simulink library "lib_cosimulation"  (Simulink 4.1.1)
undefined symbols (not defined in the file or in its folder): acc_elec_eff, acc_elec_pwr, ess2_ah_nom_fun, ess2_cap_scale, ess2_dcdc_curroutmax, ess2_dcdc_eff, ess2_dcdc_vmaxout_fun, ess2_dcdc_vminin_fun, ess2_dcdc_vminout_fun, ess2_fah_max, ess2_fah_thi, ess2_fc, ess2_init_soc, ess2_max_volts, ess2_min_volts, ess2_module_num, ess2_rnom, ess2_self_disc, ess2_sg_disc, ess2_sg_full, ess2_SOC2sg, ess2_voc, ess_ah_nom_fun, ess_cap_scale, ess_fah_max, ess_fah_thi, ess_fc, ess_init_soc, ess_max_volts, ess_min_volts, ess_module_num, ess_rnom, ess_self_disc, ess_sg_disc, ess_sg_full, ess_SOC2sg, ess_voc, fc_on, gc_cutin12, gc_cutin93, gc_eff, gc_inertia, gc_map_spd, gc_max_crrnt, gc_min_volts, gc_spd_scale, gc_t12, gc_t93, gc_tempalt, gc_user_imax12, gc_user_imax93, gc_vehicletype, mc_inertia, mc_map_spd, mc_max_crrnt, mc_min_volts, mc_spd_scale, reg_temp1, reg_temp2, reg_tempreg ... (+7)
libraries: lib_cosimulation x20
(part 1 of 2)
settings Model: LastModifiedBy=abrooker
settings Model: ModifiedHistory=|
  | [mokeefe] 22-April-2002
  | In 14V Load Control/Starter, added a memory block after the eng_on FROM tag with initial condition equal to fc_on

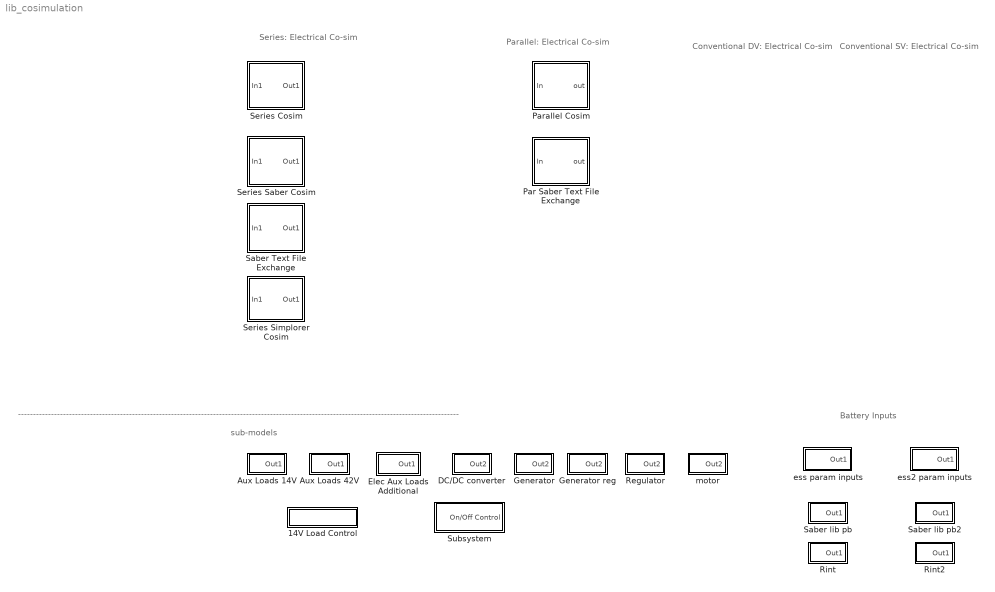
== system lib_cosimulation ==
  note: Series: Electrical Co-sim
  note: Conventional DV:
      | Electrical Co-sim
  note: ---------------------------------------------------------------------------------------------------------------------------------------------------
  note: sub-models
  note: Conventional SV:
      | Electrical Co-sim
  note: Parallel: Electrical Co-sim
  note: Battery Inputs
  14V Load Control : Subsystem
      settings: RTWFcnNameOpts=Auto  RTWFileNameOpts=Auto
  Aux Loads 14V : Subsystem
      settings: RTWFcnNameOpts=Auto  RTWFileNameOpts=Auto
  Aux Loads 42V : Subsystem
      settings: RTWFcnNameOpts=Auto  RTWFileNameOpts=Auto
  DC/DC converter : Subsystem
      settings: RTWFcnNameOpts=Auto  RTWFileNameOpts=Auto
  Elec Aux Loads Additional : Subsystem
      settings: RTWFcnNameOpts=Auto  RTWFileNameOpts=Auto
  Generator : Subsystem
      settings: RTWFcnNameOpts=Auto  RTWFileNameOpts=Auto
  Generator reg : Subsystem
      settings: RTWFcnNameOpts=Auto  RTWFileNameOpts=Auto
  Par Saber Text File Exchange : Subsystem
      settings: RTWFcnNameOpts=Auto  RTWFileNameOpts=Auto
      mask Display: image(imread('saber.bmp'))
  Parallel Cosim : Subsystem  BlockChoice=Par Saber Text File Exchange
      settings: TemplateBlock=self  MemberBlocks=Par Saber Text File Exchange  RTWFcnNameOpts=Auto  RTWFileNameOpts=Auto
  Regulator : Subsystem
      settings: RTWFcnNameOpts=Auto  RTWFileNameOpts=Auto
  Rint : Subsystem
      settings: RTWFcnNameOpts=Auto  RTWFileNameOpts=Auto
  Rint2 : Subsystem
      settings: RTWFcnNameOpts=Auto  RTWFileNameOpts=Auto
  Saber Text File Exchange : Subsystem  AncestorBlock=lib_cosimulation/SaberCosim
      settings: RTWFcnNameOpts=Auto  RTWFileNameOpts=Auto
      mask Display: image(imread('saber.bmp'))
  Saber lib pb : Subsystem
      settings: RTWFcnNameOpts=Auto  RTWFileNameOpts=Auto
  Saber lib pb2 : Subsystem
      settings: RTWFcnNameOpts=Auto  RTWFileNameOpts=Auto
  Series Cosim : Subsystem  BlockChoice=Series Saber Cosim
      settings: TemplateBlock=self  MemberBlocks=Saber Text File Exchange,Series Saber Cosim,Series Simplorer Cosim  RTWFcnNameOpts=Auto  RTWFileNameOpts=Auto
  Series Saber Cosim : Subsystem
      settings: RTWFcnNameOpts=Auto  RTWFileNameOpts=Auto
      mask Display: image(imread('saber.bmp'))
  Series Simplorer Cosim : Subsystem  AncestorBlock=lib_cosimulation/SaberCosim
      settings: RTWFcnNameOpts=Auto  RTWFileNameOpts=Auto
      mask Display: image(imread('simplorer.bmp'))
  Subsystem : Subsystem  mask{ModelName='Radio'}
      mask prompts: ModelName "Load Name (example: 'Radio')"
      settings: RTWFcnNameOpts=Auto  RTWFileNameOpts=Auto
  ess param inputs : Subsystem  BlockChoice=Rint
      settings: TemplateBlock=self  MemberBlocks=Rint,Saber lib pb  RTWFcnNameOpts=Auto  RTWFileNameOpts=Auto
  ess2 param inputs : Subsystem  BlockChoice=Rint2
      settings: TemplateBlock=self  MemberBlocks=Rint2,Saber lib pb2  RTWFcnNameOpts=Auto  RTWFileNameOpts=Auto
  motor : Subsystem
      settings: RTWFcnNameOpts=Auto  RTWFileNameOpts=Auto

== system lib_cosimulation/14V Load Control ==
  Starter : Subsystem
      settings: RTWFcnNameOpts=Auto  RTWFileNameOpts=Auto

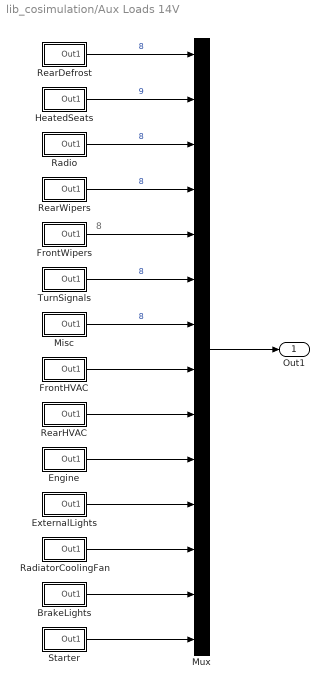
== system lib_cosimulation/Aux Loads 14V ==
  note: 8
  BrakeLights : Subsystem
      settings: RTWFcnNameOpts=Auto  RTWFileNameOpts=Auto
  Engine : Subsystem
      settings: RTWFcnNameOpts=Auto  RTWFileNameOpts=Auto
  ExternalLights : Subsystem
      settings: RTWFcnNameOpts=Auto  RTWFileNameOpts=Auto
  FrontHVAC : Subsystem
      settings: RTWFcnNameOpts=Auto  RTWFileNameOpts=Auto
  FrontWipers : Subsystem
      settings: RTWFcnNameOpts=Auto  RTWFileNameOpts=Auto
  HeatedSeats : Subsystem
      settings: RTWFcnNameOpts=Auto  RTWFileNameOpts=Auto
  Misc : Subsystem
      settings: RTWFcnNameOpts=Auto  RTWFileNameOpts=Auto
  Mux : Mux  Inputs=14
  RadiatorCoolingFan : Subsystem
      settings: RTWFcnNameOpts=Auto  RTWFileNameOpts=Auto
  Radio : Subsystem
      settings: RTWFcnNameOpts=Auto  RTWFileNameOpts=Auto
  RearDefrost : Subsystem
      settings: RTWFcnNameOpts=Auto  RTWFileNameOpts=Auto
  RearHVAC : Subsystem
      settings: RTWFcnNameOpts=Auto  RTWFileNameOpts=Auto
  RearWipers : Subsystem
      settings: RTWFcnNameOpts=Auto  RTWFileNameOpts=Auto
  Starter : Subsystem
      settings: RTWFcnNameOpts=Auto  RTWFileNameOpts=Auto
  TurnSignals : Subsystem
      settings: RTWFcnNameOpts=Auto  RTWFileNameOpts=Auto
  Out1 : Outport  Port=1
  wires:
  BrakeLights/1(Out1) -> Mux/13
  RadiatorCoolingFan/1(Out1) -> Mux/12
  ExternalLights/1(Out1) -> Mux/11
  Engine/1(Out1) -> Mux/10
  RearHVAC/1(Out1) -> Mux/9
  FrontHVAC/1(Out1) -> Mux/8
  Misc/1(Out1) -> Mux/7  "8"
  TurnSignals/1(Out1) -> Mux/6  "8"
  FrontWipers/1(Out1) -> Mux/5
  RearWipers/1(Out1) -> Mux/4  "8"
  Radio/1(Out1) -> Mux/3  "8"
  HeatedSeats/1(Out1) -> Mux/2  "9"
  RearDefrost/1(Out1) -> Mux/1  "8"
  Mux/1 -> Out1/1
  Starter/1(Out1) -> Mux/14

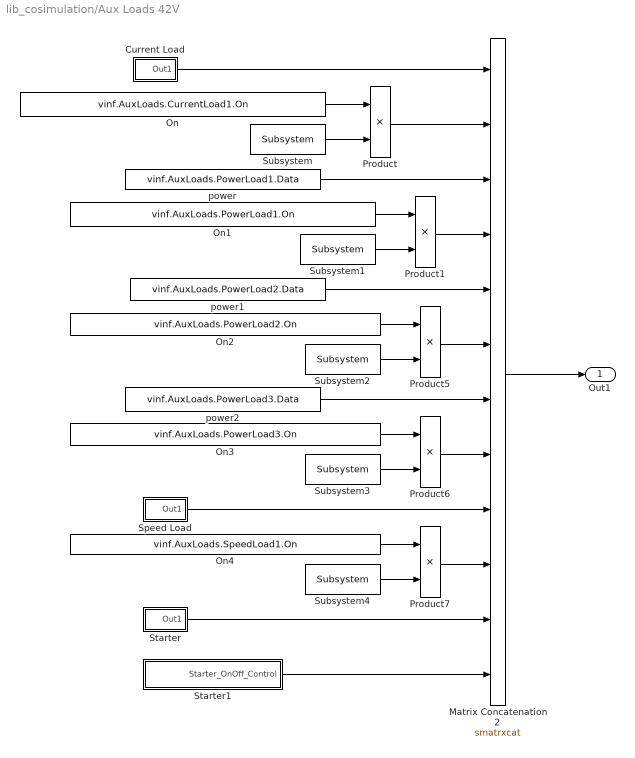
== system lib_cosimulation/Aux Loads 42V ==
  Current Load : Subsystem
      settings: RTWFcnNameOpts=Auto  RTWFileNameOpts=Auto
  Matrix Concatenation2 : S-Function  FunctionName=smatrxcat  Parameters=numInports,catMethod  PortCounts=[]  SFunctionModules=''  mask(Matrix Concatenation){numInports=12, catMethod=Horizontal}
      mask prompts: numInports "Number of inputs:"; catMethod "Concatenation method:"
      mask help: Perform horizontal or vertical concatenation. 1-D vector input signals are treated as column vectors, i.e., [Mx1] matrices. The output is always a matrix.
      mask init:
      | xy = matrxcatmask('icon');
      mask StyleString: edit,popup(Horizontal|Vertical)
      mask Display:
      | plot(xy.x,xy.y);
      | text(0.15,0.86,xy.label);
  On : Constant  Value=vinf.AuxLoads.CurrentLoad1.On
  On1 : Constant  Value=vinf.AuxLoads.PowerLoad1.On
  On2 : Constant  Value=vinf.AuxLoads.PowerLoad2.On
  On3 : Constant  Value=vinf.AuxLoads.PowerLoad3.On
  On4 : Constant  Value=vinf.AuxLoads.SpeedLoad1.On
  Product{,1,5..7} (5 alike) : Product  Inputs=2  Multiplication=Element-wise(.*)  SaturateOnIntegerOverflow=on
  Speed Load : Subsystem
      settings: RTWFcnNameOpts=Auto  RTWFileNameOpts=Auto
  Starter : Subsystem
      settings: RTWFcnNameOpts=Auto  RTWFileNameOpts=Auto
  Starter1 : Subsystem
      settings: RTWFcnNameOpts=Auto  RTWFileNameOpts=Auto
  Subsystem : lib_cosimulation/Subsystem  ModelName='CurrentLoad1'
  Subsystem1 : lib_cosimulation/Subsystem  ModelName='PowerLoad1'
  Subsystem2 : lib_cosimulation/Subsystem  ModelName='PowerLoad2'
  Subsystem3 : lib_cosimulation/Subsystem  ModelName='PowerLoad3'
  Subsystem4 : lib_cosimulation/Subsystem  ModelName='SpeedLoad1'
  power : Constant  Value=vinf.AuxLoads.PowerLoad1.Data
  power1 : Constant  Value=vinf.AuxLoads.PowerLoad2.Data
  power2 : Constant  Value=vinf.AuxLoads.PowerLoad3.Data
  Out1 : Outport  Port=1
  wires:
  power1/1 -> Matrix Concatenation2/5
  power/1 -> Matrix Concatenation2/3
  Matrix Concatenation2/1 -> Out1/1
  Speed Load/1(Out1) -> Matrix Concatenation2/9
  Current Load/1(Out1) -> Matrix Concatenation2/1
  Starter/1(Out1) -> Matrix Concatenation2/11
  power2/1 -> Matrix Concatenation2/7
  Product/1 -> Matrix Concatenation2/2
  On/1 -> Product/1
  Subsystem/1 -> Product/2
  On1/1 -> Product1/1
  Subsystem1/1 -> Product1/2
  Product1/1 -> Matrix Concatenation2/4
  Product5/1 -> Matrix Concatenation2/6
  On2/1 -> Product5/1
  Subsystem2/1 -> Product5/2
  Product6/1 -> Matrix Concatenation2/8
  On3/1 -> Product6/1
  Subsystem3/1 -> Product6/2
  Product7/1 -> Matrix Concatenation2/10
  Subsystem4/1 -> Product7/2
  On4/1 -> Product7/1
  Starter1/1(Starter_OnOff_Control) -> Matrix Concatenation2/12

== system lib_cosimulation/DC/DC converter ==
  Constant1 : Constant  Value=ess2_dcdc_eff
  Constant4 : Constant  Value=ess2_dcdc_curroutmax
  Matrix Concatenation1 : S-Function  FunctionName=smatrxcat  Parameters=numInports,catMethod  PortCounts=[]  SFunctionModules=''  mask(Matrix Concatenation){numInports=6, catMethod=Horizontal}
      mask prompts: numInports "Number of inputs:"; catMethod "Concatenation method:"
      mask help: Perform horizontal or vertical concatenation. 1-D vector input signals are treated as column vectors, i.e., [Mx1] matrices. The output is always a matrix.
      mask init:
      | xy = matrxcatmask('icon');
      mask StyleString: edit,popup(Horizontal|Vertical)
      mask Display:
      | plot(xy.x,xy.y);
      | text(0.15,0.86,xy.label);
  ess2_dcdc_vmaxout : Constant  Value=ess2_dcdc_vmaxout_fun(0)
  ess2_dcdc_vminin : Constant  Value=ess2_dcdc_vminin_fun(0)
  ess2_dcdc_vminout : Constant  Value=ess2_dcdc_vminout_fun(0)
  Out2 : Outport  Port=1
  wires:
  Matrix Concatenation1/1 -> Out2/1
  [key_on] -> Matrix Concatenation1/1
  Constant1/1 -> Matrix Concatenation1/2
  ess2_dcdc_vminout/1 -> Matrix Concatenation1/3
  ess2_dcdc_vmaxout/1 -> Matrix Concatenation1/4
  Constant4/1 -> Matrix Concatenation1/5
  ess2_dcdc_vminin/1 -> Matrix Concatenation1/6

== system lib_cosimulation/Elec Aux Loads Additional ==
  Constant : Constant  Value=acc_elec_pwr
  Product : Product  Inputs=2  Multiplication=Element-wise(.*)  SaturateOnIntegerOverflow=on
  eff : Gain  Gain=1/acc_elec_eff  Multiplication=Element-wise(K.*u)  SaturateOnIntegerOverflow=on
  Out1 : Outport  Port=1
  wires:
  Product/1 -> Out1/1
  [key_on] -> Product/1
  eff/1 -> Product/2
  Constant/1 -> eff/1

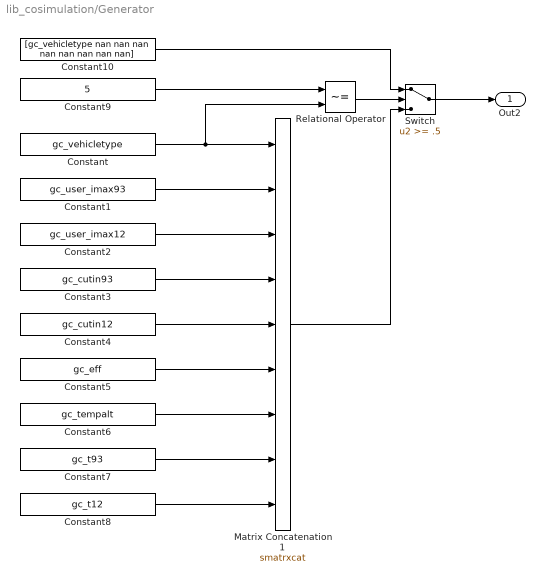
== system lib_cosimulation/Generator ==
  Constant : Constant  Value=gc_vehicletype
  Constant1 : Constant  Value=gc_user_imax93
  Constant10 : Constant  Value=[gc_vehicletype nan nan nan nan nan nan nan nan]
  Constant2 : Constant  Value=gc_user_imax12
  Constant3 : Constant  Value=gc_cutin93
  Constant4 : Constant  Value=gc_cutin12
  Constant5 : Constant  Value=gc_eff
  Constant6 : Constant  Value=gc_tempalt
  Constant7 : Constant  Value=gc_t93
  Constant8 : Constant  Value=gc_t12
  Constant9 : Constant  Value=5
  Matrix Concatenation1 : S-Function  FunctionName=smatrxcat  Parameters=numInports,catMethod  PortCounts=[]  SFunctionModules=''  mask(Matrix Concatenation){numInports=9, catMethod=Horizontal}
      mask prompts: numInports "Number of inputs:"; catMethod "Concatenation method:"
      mask help: Perform horizontal or vertical concatenation. 1-D vector input signals are treated as column vectors, i.e., [Mx1] matrices. The output is always a matrix.
      mask init:
      | xy = matrxcatmask('icon');
      mask StyleString: edit,popup(Horizontal|Vertical)
      mask Display:
      | plot(xy.x,xy.y);
      | text(0.15,0.86,xy.label);
  Relational Operator : RelationalOperator  Operator=~=
  Switch : Switch  Threshold=.5
  Out2 : Outport  Port=1
  wires:
  Constant8/1 -> Matrix Concatenation1/9
  Switch/1 -> Out2/1
  Constant1/1 -> Matrix Concatenation1/2
  Constant2/1 -> Matrix Concatenation1/3
  Constant3/1 -> Matrix Concatenation1/4
  Constant4/1 -> Matrix Concatenation1/5
  Constant5/1 -> Matrix Concatenation1/6
  Constant6/1 -> Matrix Concatenation1/7
  Constant7/1 -> Matrix Concatenation1/8
  Relational Operator/1 -> Switch/2
  Matrix Concatenation1/1 -> Switch/3
  Constant9/1 -> Relational Operator/1
  Constant/1 -> Matrix Concatenation1/1, Relational Operator/2
  Constant10/1 -> Switch/1

== system lib_cosimulation/Generator reg ==
  Constant5 : Constant  Value=gc_inertia
  Constant7 : Constant  Value=gc_max_crrnt
  Constant8 : Constant  Value=gc_min_volts
  Matrix Concatenation1 : S-Function  FunctionName=smatrxcat  Parameters=numInports,catMethod  PortCounts=[]  SFunctionModules=''  mask(Matrix Concatenation){numInports=4, catMethod=Horizontal}
      mask prompts: numInports "Number of inputs:"; catMethod "Concatenation method:"
      mask help: Perform horizontal or vertical concatenation. 1-D vector input signals are treated as column vectors, i.e., [Mx1] matrices. The output is always a matrix.
      mask init:
      | xy = matrxcatmask('icon');
      mask StyleString: edit,popup(Horizontal|Vertical)
      mask Display:
      | plot(xy.x,xy.y);
      | text(0.15,0.86,xy.label);
  max gc spd : Constant  Value=max(gc_map_spd)*gc_spd_scale
  Out2 : Outport  Port=1
  wires:
  Constant7/1 -> Matrix Concatenation1/3
  max gc spd/1 -> Matrix Concatenation1/2
  Constant5/1 -> Matrix Concatenation1/1
  Constant8/1 -> Matrix Concatenation1/4
  Matrix Concatenation1/1 -> Out2/1

== system lib_cosimulation/Par Saber Text File Exchange ==
  In : Inport  Port=1  LatchInput=off
  S-Function that calls  Saber co-simulation1 : S-Function  FunctionName=SaberCosimSfun  Parameters=vinf.tmppath,time_step,['SaberCosimIO_PAR']  PortCounts=[]  SFunctionModules=''
  out : Outport  Port=1
  wires:
  In/1 -> S-Function that calls  Saber co-simulation1/1
  S-Function that calls  Saber co-simulation1/1 -> out/1

== system lib_cosimulation/Parallel Cosim ==
  In : Inport  Port=1  LatchInput=off
  Par Saber Text File Exchange : lib_cosimulation/Par Saber Text File Exchange
  out : Outport  Port=1
  wires:
  In/1 -> Par Saber Text File Exchange/1
  Par Saber Text File Exchange/1 -> out/1

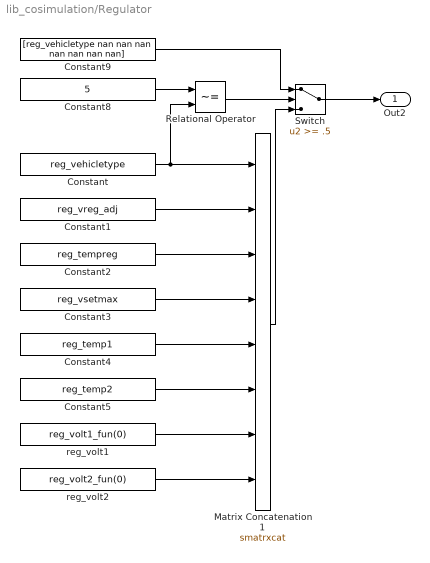
== system lib_cosimulation/Regulator ==
  Constant : Constant  Value=reg_vehicletype
  Constant1 : Constant  Value=reg_vreg_adj
  Constant2 : Constant  Value=reg_tempreg
  Constant3 : Constant  Value=reg_vsetmax
  Constant4 : Constant  Value=reg_temp1
  Constant5 : Constant  Value=reg_temp2
  Constant8 : Constant  Value=5
  Constant9 : Constant  Value=[reg_vehicletype nan nan nan nan nan nan nan]
  Matrix Concatenation1 : S-Function  FunctionName=smatrxcat  Parameters=numInports,catMethod  PortCounts=[]  SFunctionModules=''  mask(Matrix Concatenation){numInports=8, catMethod=Horizontal}
      mask prompts: numInports "Number of inputs:"; catMethod "Concatenation method:"
      mask help: Perform horizontal or vertical concatenation. 1-D vector input signals are treated as column vectors, i.e., [Mx1] matrices. The output is always a matrix.
      mask init:
      | xy = matrxcatmask('icon');
      mask StyleString: edit,popup(Horizontal|Vertical)
      mask Display:
      | plot(xy.x,xy.y);
      | text(0.15,0.86,xy.label);
  Relational Operator : RelationalOperator  Operator=~=
  Switch : Switch  Threshold=.5
  reg_volt1 : Constant  Value=reg_volt1_fun(0)
  reg_volt2 : Constant  Value=reg_volt2_fun(0)
  Out2 : Outport  Port=1
  wires:
  Constant/1 -> Matrix Concatenation1/1, Relational Operator/2
  Constant1/1 -> Matrix Concatenation1/2
  Constant2/1 -> Matrix Concatenation1/3
  Constant3/1 -> Matrix Concatenation1/4
  Constant4/1 -> Matrix Concatenation1/5
  Constant5/1 -> Matrix Concatenation1/6
  reg_volt1/1 -> Matrix Concatenation1/7
  reg_volt2/1 -> Matrix Concatenation1/8
  Switch/1 -> Out2/1
  Matrix Concatenation1/1 -> Switch/3
  Relational Operator/1 -> Switch/2
  Constant8/1 -> Relational Operator/1
  Constant9/1 -> Switch/1

== system lib_cosimulation/Rint ==
  Matrix Concatenation1 : S-Function  FunctionName=smatrxcat  Parameters=numInports,catMethod  PortCounts=[]  SFunctionModules=''  mask(Matrix Concatenation){numInports=4, catMethod=Horizontal}
      mask prompts: numInports "Number of inputs:"; catMethod "Concatenation method:"
      mask help: Perform horizontal or vertical concatenation. 1-D vector input signals are treated as column vectors, i.e., [Mx1] matrices. The output is always a matrix.
      mask init:
      | xy = matrxcatmask('icon');
      mask StyleString: edit,popup(Horizontal|Vertical)
      mask Display:
      | plot(xy.x,xy.y);
      | text(0.15,0.86,xy.label);
  ess_init_soc : Constant  Value=ess_max_volts  VectorParams1D=off
  ess_init_soc1 : Constant  Value=ess_init_soc
  ess_init_soc2 : Constant  Value=ess_module_num  VectorParams1D=off
  ess_init_soc3 : Constant  Value=ess_min_volts  VectorParams1D=off
  Out1 : Outport  Port=1
  wires:
  ess_init_soc1/1 -> Matrix Concatenation1/4
  ess_init_soc3/1 -> Matrix Concatenation1/3
  ess_init_soc2/1 -> Matrix Concatenation1/2
  Matrix Concatenation1/1 -> Out1/1
  ess_init_soc/1 -> Matrix Concatenation1/1

== system lib_cosimulation/Rint2 ==
  Matrix Concatenation1 : S-Function  FunctionName=smatrxcat  Parameters=numInports,catMethod  PortCounts=[]  SFunctionModules=''  mask(Matrix Concatenation){numInports=4, catMethod=Horizontal}
      mask prompts: numInports "Number of inputs:"; catMethod "Concatenation method:"
      mask help: Perform horizontal or vertical concatenation. 1-D vector input signals are treated as column vectors, i.e., [Mx1] matrices. The output is always a matrix.
      mask init:
      | xy = matrxcatmask('icon');
      mask StyleString: edit,popup(Horizontal|Vertical)
      mask Display:
      | plot(xy.x,xy.y);
      | text(0.15,0.86,xy.label);
  ess_init_soc : Constant  Value=ess2_max_volts  VectorParams1D=off
  ess_init_soc1 : Constant  Value=ess2_init_soc
  ess_init_soc2 : Constant  Value=ess2_module_num  VectorParams1D=off
  ess_init_soc3 : Constant  Value=ess2_min_volts  VectorParams1D=off
  Out1 : Outport  Port=1
  wires:
  ess_init_soc/1 -> Matrix Concatenation1/1
  Matrix Concatenation1/1 -> Out1/1
  ess_init_soc2/1 -> Matrix Concatenation1/2
  ess_init_soc3/1 -> Matrix Concatenation1/3
  ess_init_soc1/1 -> Matrix Concatenation1/4

== system lib_cosimulation/Saber Text File Exchange ==
  In1 : Inport  Port=1  LatchInput=off
  S-Function that calls  Saber co-simulation inputs: engine speed (rad/s) load parameters outputs: accessory power model outputs (e.g. pwrs)2 : S-Function  FunctionName=SaberCosimSfun  Parameters=vinf.tmppath,time_step,['SaberCosimIO_SER']  PortCounts=[]  SFunctionModules=''
  Out1 : Outport  Port=1
  wires:
  S-Function that calls  Saber co-simulation inputs: engine speed (rad/s) load parameters outputs: accessory power model outputs (e.g. pwrs)2/1 -> Out1/1
  In1/1 -> S-Function that calls  Saber co-simulation inputs: engine speed (rad/s) load parameters outputs: accessory power model outputs (e.g. pwrs)2/1

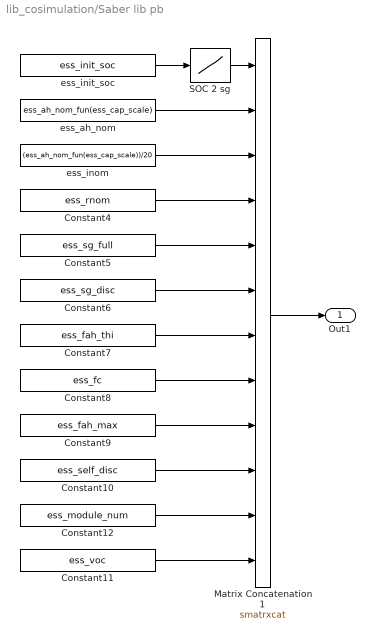
== system lib_cosimulation/Saber lib pb ==
  Constant10 : Constant  Value=ess_self_disc
  Constant11 : Constant  Value=ess_voc
  Constant12 : Constant  Value=ess_module_num
  Constant4 : Constant  Value=ess_rnom
  Constant5 : Constant  Value=ess_sg_full
  Constant6 : Constant  Value=ess_sg_disc
  Constant7 : Constant  Value=ess_fah_thi
  Constant8 : Constant  Value=ess_fc
  Constant9 : Constant  Value=ess_fah_max
  Matrix Concatenation1 : S-Function  FunctionName=smatrxcat  Parameters=numInports,catMethod  PortCounts=[]  SFunctionModules=''  mask(Matrix Concatenation){numInports=12, catMethod=Horizontal}
      mask prompts: numInports "Number of inputs:"; catMethod "Concatenation method:"
      mask help: Perform horizontal or vertical concatenation. 1-D vector input signals are treated as column vectors, i.e., [Mx1] matrices. The output is always a matrix.
      mask init:
      | xy = matrxcatmask('icon');
      mask StyleString: edit,popup(Horizontal|Vertical)
      mask Display:
      | plot(xy.x,xy.y);
      | text(0.15,0.86,xy.label);
  SOC 2 sg : Lookup  InputValues=ess_SOC2sg(:,1)  OutputValues=ess_SOC2sg(:,2)
  ess_ah_nom : Constant  Value=ess_ah_nom_fun(ess_cap_scale)
  ess_init_soc : Constant  Value=ess_init_soc
  ess_inom : Constant  Value=(ess_ah_nom_fun(ess_cap_scale))/20
  Out1 : Outport  Port=1
  wires:
  Constant11/1 -> Matrix Concatenation1/12
  Constant12/1 -> Matrix Concatenation1/11
  Matrix Concatenation1/1 -> Out1/1
  ess_ah_nom/1 -> Matrix Concatenation1/2
  ess_inom/1 -> Matrix Concatenation1/3
  Constant4/1 -> Matrix Concatenation1/4
  Constant5/1 -> Matrix Concatenation1/5
  Constant6/1 -> Matrix Concatenation1/6
  Constant7/1 -> Matrix Concatenation1/7
  Constant8/1 -> Matrix Concatenation1/8
  Constant9/1 -> Matrix Concatenation1/9
  Constant10/1 -> Matrix Concatenation1/10
  ess_init_soc/1 -> SOC 2 sg/1
  SOC 2 sg/1 -> Matrix Concatenation1/1

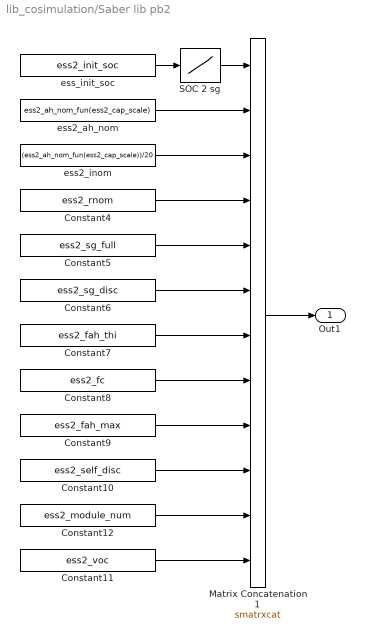
== system lib_cosimulation/Saber lib pb2 ==
  Constant10 : Constant  Value=ess2_self_disc
  Constant11 : Constant  Value=ess2_voc
  Constant12 : Constant  Value=ess2_module_num
  Constant4 : Constant  Value=ess2_rnom
  Constant5 : Constant  Value=ess2_sg_full
  Constant6 : Constant  Value=ess2_sg_disc
  Constant7 : Constant  Value=ess2_fah_thi
  Constant8 : Constant  Value=ess2_fc
  Constant9 : Constant  Value=ess2_fah_max
  Matrix Concatenation1 : S-Function  FunctionName=smatrxcat  Parameters=numInports,catMethod  PortCounts=[]  SFunctionModules=''  mask(Matrix Concatenation){numInports=12, catMethod=Horizontal}
      mask prompts: numInports "Number of inputs:"; catMethod "Concatenation method:"
      mask help: Perform horizontal or vertical concatenation. 1-D vector input signals are treated as column vectors, i.e., [Mx1] matrices. The output is always a matrix.
      mask init:
      | xy = matrxcatmask('icon');
      mask StyleString: edit,popup(Horizontal|Vertical)
      mask Display:
      | plot(xy.x,xy.y);
      | text(0.15,0.86,xy.label);
  SOC 2 sg : Lookup  InputValues=ess2_SOC2sg(:,1)  OutputValues=ess2_SOC2sg(:,2)
  ess2_ah_nom : Constant  Value=ess2_ah_nom_fun(ess2_cap_scale)
  ess2_inom : Constant  Value=(ess2_ah_nom_fun(ess2_cap_scale))/20
  ess_init_soc : Constant  Value=ess2_init_soc
  Out1 : Outport  Port=1
  wires:
  Constant11/1 -> Matrix Concatenation1/12
  Constant12/1 -> Matrix Concatenation1/11
  Matrix Concatenation1/1 -> Out1/1
  ess2_ah_nom/1 -> Matrix Concatenation1/2
  ess2_inom/1 -> Matrix Concatenation1/3
  Constant4/1 -> Matrix Concatenation1/4
  Constant5/1 -> Matrix Concatenation1/5
  Constant6/1 -> Matrix Concatenation1/6
  Constant7/1 -> Matrix Concatenation1/7
  Constant8/1 -> Matrix Concatenation1/8
  Constant9/1 -> Matrix Concatenation1/9
  Constant10/1 -> Matrix Concatenation1/10
  ess_init_soc/1 -> SOC 2 sg/1
  SOC 2 sg/1 -> Matrix Concatenation1/1

== system lib_cosimulation/Series Cosim ==
  In1 : Inport  Port=1  LatchInput=off
  Series Saber Cosim : lib_cosimulation/Series Saber Cosim
  Out1 : Outport  Port=1
  wires:
  In1/1 -> Series Saber Cosim/1
  Series Saber Cosim/1 -> Out1/1

== system lib_cosimulation/Series Saber Cosim ==
  In1 : Inport  Port=1  LatchInput=off
  Out1 : Outport  Port=1
  wires:
  ? -> Out1/1
  In1/1 -> ?

== system lib_cosimulation/Series Simplorer Cosim ==
  In1 : Inport  Port=1  LatchInput=off
  Demux : Demux  Outputs=6  BusSelectionMode=off
  Mux : Mux  Inputs=2
  Out1 : Outport  Port=1
  wires:
  In1/1 -> Demux/1
  Mux/1 -> Out1/1

== system lib_cosimulation/Subsystem ==
  Load On/Off : Switch  Threshold=.5
  On/Off checkbox : Gain  Gain=vinf.AuxLoadsOn  Multiplication=Element-wise(K.*u)  SaturateOnIntegerOverflow=on
  Product : Product  Inputs=2  Multiplication=Element-wise(.*)  SaturateOnIntegerOverflow=on
  Regular Cycles (1) or Toggle On Off (0) : Constant  Value=strcmp(evalin('base',['vinf.AuxLoads.',ModelName,'.OnOffInfo.Type']),'RegularCycles')
  Subsystem : Subsystem
      settings: RTWFcnNameOpts=Auto  RTWFileNameOpts=Auto
  Subsystem1 : Subsystem
      settings: RTWFcnNameOpts=Auto  RTWFileNameOpts=Auto
  On/Off Control : Outport  Port=1
  wires:
  Subsystem1/1(Toggle On/Off) -> Load On/Off/3
  Subsystem/1(Reg Cycle On/Off) -> Load On/Off/1
  Regular Cycles (1) or Toggle On Off (0)/1 -> Load On/Off/2
  Product/1 -> On/Off checkbox/1
  Load On/Off/1 -> Product/1
  [key_on] -> Product/2
  On/Off checkbox/1 -> On/Off Control/1

== system lib_cosimulation/ess param inputs ==
  Rint : lib_cosimulation/Rint
      settings: RTWFcnNameOpts=Auto  RTWFileNameOpts=Auto
  Out1 : Outport  Port=1
  wires:
  Rint/1 -> Out1/1

== system lib_cosimulation/ess2 param inputs ==
  Rint2 : lib_cosimulation/Rint
      settings: RTWFcnNameOpts=Auto  RTWFileNameOpts=Auto
  Out1 : Outport  Port=1
  wires:
  Rint2/1 -> Out1/1

== system lib_cosimulation/motor ==
  Constant5 : Constant  Value=mc_inertia
  Constant7 : Constant  Value=mc_max_crrnt
  Constant8 : Constant  Value=mc_min_volts
  Matrix Concatenation1 : S-Function  FunctionName=smatrxcat  Parameters=numInports,catMethod  PortCounts=[]  SFunctionModules=''  mask(Matrix Concatenation){numInports=4, catMethod=Horizontal}
      mask prompts: numInports "Number of inputs:"; catMethod "Concatenation method:"
      mask help: Perform horizontal or vertical concatenation. 1-D vector input signals are treated as column vectors, i.e., [Mx1] matrices. The output is always a matrix.
      mask init:
      | xy = matrxcatmask('icon');
      mask StyleString: edit,popup(Horizontal|Vertical)
      mask Display:
      | plot(xy.x,xy.y);
      | text(0.15,0.86,xy.label);
  max gc spd : Constant  Value=max(mc_map_spd)*mc_spd_scale
  Out2 : Outport  Port=1
  wires:
  Matrix Concatenation1/1 -> Out2/1
  Constant8/1 -> Matrix Concatenation1/4
  Constant5/1 -> Matrix Concatenation1/1
  max gc spd/1 -> Matrix Concatenation1/2
  Constant7/1 -> Matrix Concatenation1/3

== system lib_cosimulation/14V Load Control/Starter ==
  14 V : Constant  Value=vinf.AuxLoads.Starter.V14
  Hit  Crossing : HitCross  HitCrossingOffset=0  HitCrossingDirection=rising  ShowOutputPort=on
  Memory : Memory  X0=fc_on  InheritSampleTime=off
      settings: RTWStateStorageClass=Auto
  On : Constant  Value=vinf.AuxLoads.Starter.On
  Product1 : Product  Inputs=4  Multiplication=Element-wise(.*)  SaturateOnIntegerOverflow=on
  Subsystem : Subsystem
      settings: RTWFcnNameOpts=Auto  RTWFileNameOpts=Auto
  Starter_OnOff_Control : Outport  Port=1
  wires:
  Memory/1 -> Hit  Crossing/1
  Hit  Crossing/1 -> Subsystem/1(In1)
  [engine_on] -> Memory/1
  [time] -> Subsystem/2(In2)
  [key_on] -> Product1/4
  On/1 -> Product1/1
  Product1/1 -> Starter_OnOff_Control/1
  Subsystem/1(Out1) -> Product1/3
  14 V/1 -> Product1/2

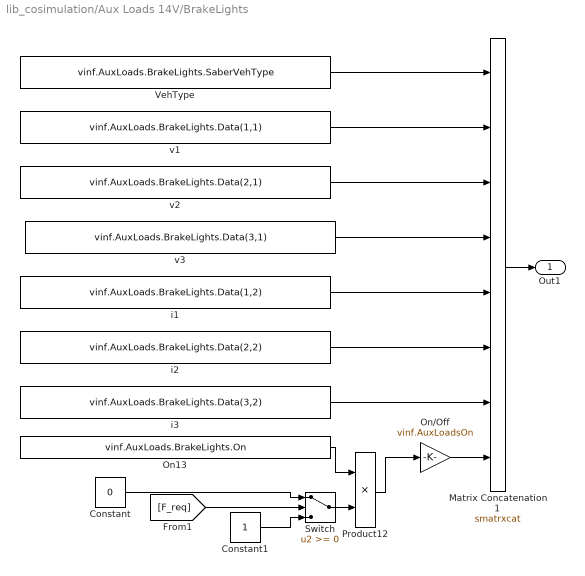
== system lib_cosimulation/Aux Loads 14V/BrakeLights ==
  Constant : Constant  Value=0
  Constant1 : Constant  Value=1
  Matrix Concatenation1 : S-Function  FunctionName=smatrxcat  Parameters=numInports,catMethod  PortCounts=[]  SFunctionModules=''  mask(Matrix Concatenation){numInports=8, catMethod=Horizontal}
      mask prompts: numInports "Number of inputs:"; catMethod "Concatenation method:"
      mask help: Perform horizontal or vertical concatenation. 1-D vector input signals are treated as column vectors, i.e., [Mx1] matrices. The output is always a matrix.
      mask init:
      | xy = matrxcatmask('icon');
      mask StyleString: edit,popup(Horizontal|Vertical)
      mask Display:
      | plot(xy.x,xy.y);
      | text(0.15,0.86,xy.label);
  On/Off : Gain  Gain=vinf.AuxLoadsOn  Multiplication=Element-wise(K.*u)  SaturateOnIntegerOverflow=on
  On13 : Constant  Value=vinf.AuxLoads.BrakeLights.On
  Product12 : Product  Inputs=2  Multiplication=Element-wise(.*)  SaturateOnIntegerOverflow=on
  Switch : Switch  Threshold=0
  VehType : Constant  Value=vinf.AuxLoads.BrakeLights.SaberVehType
  i1 : Constant  Value=vinf.AuxLoads.BrakeLights.Data(1,2)
  i2 : Constant  Value=vinf.AuxLoads.BrakeLights.Data(2,2)
  i3 : Constant  Value=vinf.AuxLoads.BrakeLights.Data(3,2)
  v1 : Constant  Value=vinf.AuxLoads.BrakeLights.Data(1,1)
  v2 : Constant  Value=vinf.AuxLoads.BrakeLights.Data(2,1)
  v3 : Constant  Value=vinf.AuxLoads.BrakeLights.Data(3,1)
  Out1 : Outport  Port=1
  wires:
  VehType/1 -> Matrix Concatenation1/1
  i3/1 -> Matrix Concatenation1/7
  i2/1 -> Matrix Concatenation1/6
  i1/1 -> Matrix Concatenation1/5
  v3/1 -> Matrix Concatenation1/4
  v2/1 -> Matrix Concatenation1/3
  v1/1 -> Matrix Concatenation1/2
  Matrix Concatenation1/1 -> Out1/1
  Product12/1 -> On/Off/1
  On13/1 -> Product12/1
  Constant/1 -> Switch/1
  [F_req] -> Switch/2
  Constant1/1 -> Switch/3
  Switch/1 -> Product12/2
  On/Off/1 -> Matrix Concatenation1/8

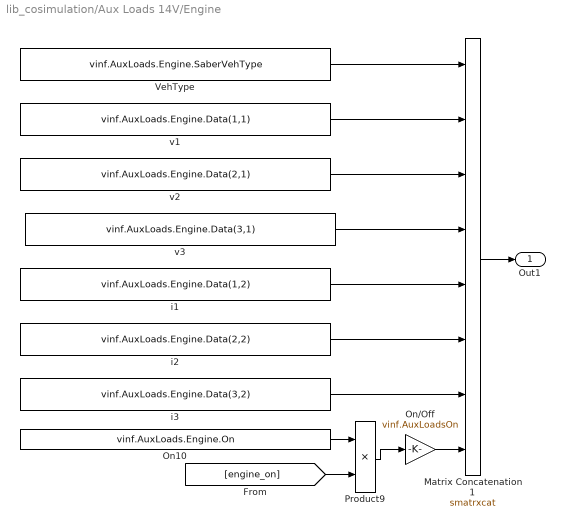
== system lib_cosimulation/Aux Loads 14V/Engine ==
  Matrix Concatenation1 : S-Function  FunctionName=smatrxcat  Parameters=numInports,catMethod  PortCounts=[]  SFunctionModules=''  mask(Matrix Concatenation){numInports=8, catMethod=Horizontal}
      mask prompts: numInports "Number of inputs:"; catMethod "Concatenation method:"
      mask help: Perform horizontal or vertical concatenation. 1-D vector input signals are treated as column vectors, i.e., [Mx1] matrices. The output is always a matrix.
      mask init:
      | xy = matrxcatmask('icon');
      mask StyleString: edit,popup(Horizontal|Vertical)
      mask Display:
      | plot(xy.x,xy.y);
      | text(0.15,0.86,xy.label);
  On/Off : Gain  Gain=vinf.AuxLoadsOn  Multiplication=Element-wise(K.*u)  SaturateOnIntegerOverflow=on
  On10 : Constant  Value=vinf.AuxLoads.Engine.On
  Product9 : Product  Inputs=2  Multiplication=Element-wise(.*)  SaturateOnIntegerOverflow=on
  VehType : Constant  Value=vinf.AuxLoads.Engine.SaberVehType
  i1 : Constant  Value=vinf.AuxLoads.Engine.Data(1,2)
  i2 : Constant  Value=vinf.AuxLoads.Engine.Data(2,2)
  i3 : Constant  Value=vinf.AuxLoads.Engine.Data(3,2)
  v1 : Constant  Value=vinf.AuxLoads.Engine.Data(1,1)
  v2 : Constant  Value=vinf.AuxLoads.Engine.Data(2,1)
  v3 : Constant  Value=vinf.AuxLoads.Engine.Data(3,1)
  Out1 : Outport  Port=1
  wires:
  i3/1 -> Matrix Concatenation1/7
  i2/1 -> Matrix Concatenation1/6
  i1/1 -> Matrix Concatenation1/5
  v3/1 -> Matrix Concatenation1/4
  v2/1 -> Matrix Concatenation1/3
  v1/1 -> Matrix Concatenation1/2
  Matrix Concatenation1/1 -> Out1/1
  VehType/1 -> Matrix Concatenation1/1
  Product9/1 -> On/Off/1
  On10/1 -> Product9/1
  [engine_on] -> Product9/2
  On/Off/1 -> Matrix Concatenation1/8

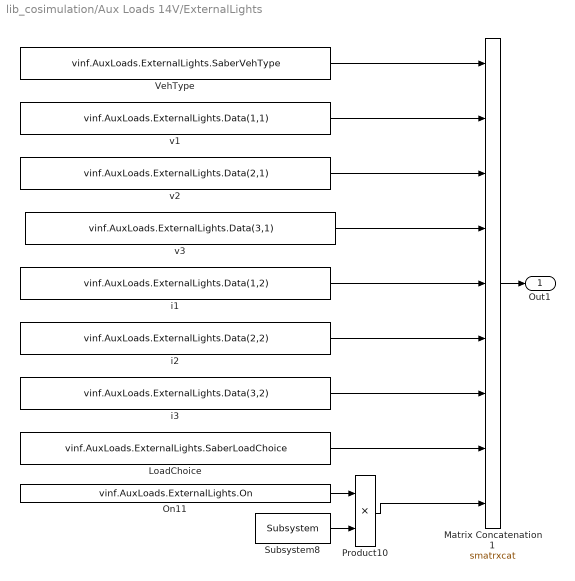
== system lib_cosimulation/Aux Loads 14V/ExternalLights ==
  LoadChoice : Constant  Value=vinf.AuxLoads.ExternalLights.SaberLoadChoice
  Matrix Concatenation1 : S-Function  FunctionName=smatrxcat  Parameters=numInports,catMethod  PortCounts=[]  SFunctionModules=''  mask(Matrix Concatenation){numInports=9, catMethod=Horizontal}
      mask prompts: numInports "Number of inputs:"; catMethod "Concatenation method:"
      mask help: Perform horizontal or vertical concatenation. 1-D vector input signals are treated as column vectors, i.e., [Mx1] matrices. The output is always a matrix.
      mask init:
      | xy = matrxcatmask('icon');
      mask StyleString: edit,popup(Horizontal|Vertical)
      mask Display:
      | plot(xy.x,xy.y);
      | text(0.15,0.86,xy.label);
  On11 : Constant  Value=vinf.AuxLoads.ExternalLights.On
  Product10 : Product  Inputs=2  Multiplication=Element-wise(.*)  SaturateOnIntegerOverflow=on
  Subsystem8 : lib_cosimulation/Subsystem  ModelName='ExternalLights'
  VehType : Constant  Value=vinf.AuxLoads.ExternalLights.SaberVehType
  i1 : Constant  Value=vinf.AuxLoads.ExternalLights.Data(1,2)
  i2 : Constant  Value=vinf.AuxLoads.ExternalLights.Data(2,2)
  i3 : Constant  Value=vinf.AuxLoads.ExternalLights.Data(3,2)
  v1 : Constant  Value=vinf.AuxLoads.ExternalLights.Data(1,1)
  v2 : Constant  Value=vinf.AuxLoads.ExternalLights.Data(2,1)
  v3 : Constant  Value=vinf.AuxLoads.ExternalLights.Data(3,1)
  Out1 : Outport  Port=1
  wires:
  LoadChoice/1 -> Matrix Concatenation1/8
  i3/1 -> Matrix Concatenation1/7
  i2/1 -> Matrix Concatenation1/6
  i1/1 -> Matrix Concatenation1/5
  v3/1 -> Matrix Concatenation1/4
  v2/1 -> Matrix Concatenation1/3
  v1/1 -> Matrix Concatenation1/2
  VehType/1 -> Matrix Concatenation1/1
  Matrix Concatenation1/1 -> Out1/1
  Product10/1 -> Matrix Concatenation1/9
  On11/1 -> Product10/1
  Subsystem8/1 -> Product10/2

== system lib_cosimulation/Aux Loads 14V/FrontHVAC ==
  LoadChoice : Constant  Value=vinf.AuxLoads.FrontHVAC.SaberLoadChoice
  Matrix Concatenation1 : S-Function  FunctionName=smatrxcat  Parameters=numInports,catMethod  PortCounts=[]  SFunctionModules=''  mask(Matrix Concatenation){numInports=9, catMethod=Horizontal}
      mask prompts: numInports "Number of inputs:"; catMethod "Concatenation method:"
      mask help: Perform horizontal or vertical concatenation. 1-D vector input signals are treated as column vectors, i.e., [Mx1] matrices. The output is always a matrix.
      mask init:
      | xy = matrxcatmask('icon');
      mask StyleString: edit,popup(Horizontal|Vertical)
      mask Display:
      | plot(xy.x,xy.y);
      | text(0.15,0.86,xy.label);
  On8 : Constant  Value=vinf.AuxLoads.FrontHVAC.On
  Product7 : Product  Inputs=2  Multiplication=Element-wise(.*)  SaturateOnIntegerOverflow=on
  Subsystem6 : lib_cosimulation/Subsystem  ModelName='FrontHVAC'
  VehType : Constant  Value=vinf.AuxLoads.FrontHVAC.SaberVehType
  i1 : Constant  Value=vinf.AuxLoads.FrontHVAC.Data(1,2)
  i2 : Constant  Value=vinf.AuxLoads.FrontHVAC.Data(2,2)
  i3 : Constant  Value=vinf.AuxLoads.FrontHVAC.Data(3,2)
  v1 : Constant  Value=vinf.AuxLoads.FrontHVAC.Data(1,1)
  v2 : Constant  Value=vinf.AuxLoads.FrontHVAC.Data(2,1)
  v3 : Constant  Value=vinf.AuxLoads.FrontHVAC.Data(3,1)
  Out1 : Outport  Port=1
  wires:
  LoadChoice/1 -> Matrix Concatenation1/8
  i3/1 -> Matrix Concatenation1/7
  i2/1 -> Matrix Concatenation1/6
  i1/1 -> Matrix Concatenation1/5
  v3/1 -> Matrix Concatenation1/4
  v2/1 -> Matrix Concatenation1/3
  v1/1 -> Matrix Concatenation1/2
  VehType/1 -> Matrix Concatenation1/1
  Matrix Concatenation1/1 -> Out1/1
  Product7/1 -> Matrix Concatenation1/9
  On8/1 -> Product7/1
  Subsystem6/1 -> Product7/2

== system lib_cosimulation/Aux Loads 14V/FrontWipers ==
  Matrix Concatenation1 : S-Function  FunctionName=smatrxcat  Parameters=numInports,catMethod  PortCounts=[]  SFunctionModules=''  mask(Matrix Concatenation){numInports=8, catMethod=Horizontal}
      mask prompts: numInports "Number of inputs:"; catMethod "Concatenation method:"
      mask help: Perform horizontal or vertical concatenation. 1-D vector input signals are treated as column vectors, i.e., [Mx1] matrices. The output is always a matrix.
      mask init:
      | xy = matrxcatmask('icon');
      mask StyleString: edit,popup(Horizontal|Vertical)
      mask Display:
      | plot(xy.x,xy.y);
      | text(0.15,0.86,xy.label);
  On5 : Constant  Value=vinf.AuxLoads.FrontWipers.On
  Product5 : Product  Inputs=2  Multiplication=Element-wise(.*)  SaturateOnIntegerOverflow=on
  Subsystem3 : lib_cosimulation/Subsystem  ModelName='FrontWipers'
  VehType : Constant  Value=vinf.AuxLoads.FrontWipers.SaberVehType
  i1 : Constant  Value=vinf.AuxLoads.FrontWipers.Data(1,2)
  i2 : Constant  Value=vinf.AuxLoads.FrontWipers.Data(2,2)
  i3 : Constant  Value=vinf.AuxLoads.FrontWipers.Data(3,2)
  v1 : Constant  Value=vinf.AuxLoads.FrontWipers.Data(1,1)
  v2 : Constant  Value=vinf.AuxLoads.FrontWipers.Data(2,1)
  v3 : Constant  Value=vinf.AuxLoads.FrontWipers.Data(3,1)
  Out1 : Outport  Port=1
  wires:
  VehType/1 -> Matrix Concatenation1/1
  i2/1 -> Matrix Concatenation1/6
  i3/1 -> Matrix Concatenation1/7
  i1/1 -> Matrix Concatenation1/5
  v3/1 -> Matrix Concatenation1/4
  v2/1 -> Matrix Concatenation1/3
  v1/1 -> Matrix Concatenation1/2
  Matrix Concatenation1/1 -> Out1/1
  Product5/1 -> Matrix Concatenation1/8
  On5/1 -> Product5/1
  Subsystem3/1 -> Product5/2

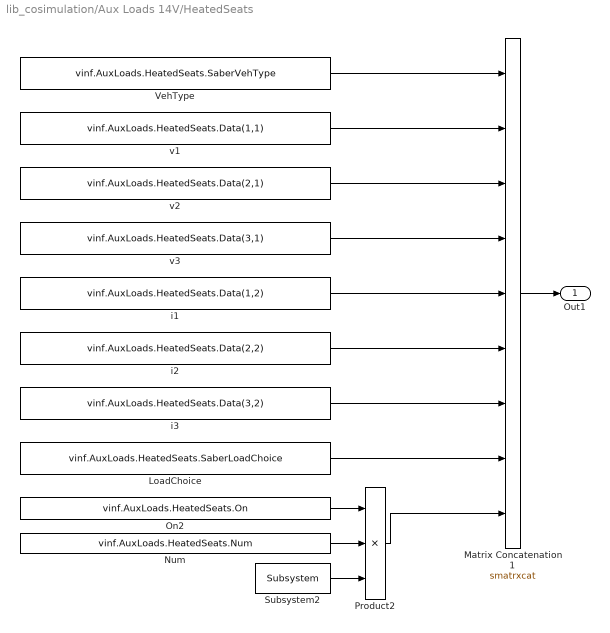
== system lib_cosimulation/Aux Loads 14V/HeatedSeats ==
  LoadChoice : Constant  Value=vinf.AuxLoads.HeatedSeats.SaberLoadChoice
  Matrix Concatenation1 : S-Function  FunctionName=smatrxcat  Parameters=numInports,catMethod  PortCounts=[]  SFunctionModules=''  mask(Matrix Concatenation){numInports=9, catMethod=Horizontal}
      mask prompts: numInports "Number of inputs:"; catMethod "Concatenation method:"
      mask help: Perform horizontal or vertical concatenation. 1-D vector input signals are treated as column vectors, i.e., [Mx1] matrices. The output is always a matrix.
      mask init:
      | xy = matrxcatmask('icon');
      mask StyleString: edit,popup(Horizontal|Vertical)
      mask Display:
      | plot(xy.x,xy.y);
      | text(0.15,0.86,xy.label);
  Num : Constant  Value=vinf.AuxLoads.HeatedSeats.Num
  On2 : Constant  Value=vinf.AuxLoads.HeatedSeats.On
  Product2 : Product  Inputs=3  Multiplication=Element-wise(.*)  SaturateOnIntegerOverflow=on
  Subsystem2 : lib_cosimulation/Subsystem  ModelName='HeatedSeats'
  VehType : Constant  Value=vinf.AuxLoads.HeatedSeats.SaberVehType
  i1 : Constant  Value=vinf.AuxLoads.HeatedSeats.Data(1,2)
  i2 : Constant  Value=vinf.AuxLoads.HeatedSeats.Data(2,2)
  i3 : Constant  Value=vinf.AuxLoads.HeatedSeats.Data(3,2)
  v1 : Constant  Value=vinf.AuxLoads.HeatedSeats.Data(1,1)
  v2 : Constant  Value=vinf.AuxLoads.HeatedSeats.Data(2,1)
  v3 : Constant  Value=vinf.AuxLoads.HeatedSeats.Data(3,1)
  Out1 : Outport  Port=1
  wires:
  Matrix Concatenation1/1 -> Out1/1
  LoadChoice/1 -> Matrix Concatenation1/8
  v1/1 -> Matrix Concatenation1/2
  v2/1 -> Matrix Concatenation1/3
  v3/1 -> Matrix Concatenation1/4
  i1/1 -> Matrix Concatenation1/5
  i2/1 -> Matrix Concatenation1/6
  i3/1 -> Matrix Concatenation1/7
  VehType/1 -> Matrix Concatenation1/1
  Product2/1 -> Matrix Concatenation1/9
  On2/1 -> Product2/1
  Num/1 -> Product2/2
  Subsystem2/1 -> Product2/3

== system lib_cosimulation/Aux Loads 14V/Misc ==
  Matrix Concatenation1 : S-Function  FunctionName=smatrxcat  Parameters=numInports,catMethod  PortCounts=[]  SFunctionModules=''  mask(Matrix Concatenation){numInports=8, catMethod=Horizontal}
      mask prompts: numInports "Number of inputs:"; catMethod "Concatenation method:"
      mask help: Perform horizontal or vertical concatenation. 1-D vector input signals are treated as column vectors, i.e., [Mx1] matrices. The output is always a matrix.
      mask init:
      | xy = matrxcatmask('icon');
      mask StyleString: edit,popup(Horizontal|Vertical)
      mask Display:
      | plot(xy.x,xy.y);
      | text(0.15,0.86,xy.label);
  On/Off : Gain  Gain=vinf.AuxLoadsOn  Multiplication=Element-wise(K.*u)  SaturateOnIntegerOverflow=on
  On7 : Constant  Value=vinf.AuxLoads.Misc.On
  Product : Product  Inputs=2  Multiplication=Element-wise(.*)  SaturateOnIntegerOverflow=on
  VehType : Constant  Value=vinf.AuxLoads.Misc.SaberVehType
  i1 : Constant  Value=vinf.AuxLoads.Misc.Data(1,2)
  i2 : Constant  Value=vinf.AuxLoads.Misc.Data(2,2)
  i3 : Constant  Value=vinf.AuxLoads.Misc.Data(3,2)
  v1 : Constant  Value=vinf.AuxLoads.Misc.Data(1,1)
  v2 : Constant  Value=vinf.AuxLoads.Misc.Data(2,1)
  v3 : Constant  Value=vinf.AuxLoads.Misc.Data(3,1)
  Out1 : Outport  Port=1
  wires:
  VehType/1 -> Matrix Concatenation1/1
  i3/1 -> Matrix Concatenation1/7
  i2/1 -> Matrix Concatenation1/6
  i1/1 -> Matrix Concatenation1/5
  v3/1 -> Matrix Concatenation1/4
  v2/1 -> Matrix Concatenation1/3
  v1/1 -> Matrix Concatenation1/2
  Matrix Concatenation1/1 -> Out1/1
  Product/1 -> On/Off/1
  On7/1 -> Product/1
  [key_on] -> Product/2
  On/Off/1 -> Matrix Concatenation1/8

== system lib_cosimulation/Aux Loads 14V/RadiatorCoolingFan ==
  LoadChoice : Constant  Value=vinf.AuxLoads.RadiatorCoolingFan.SaberLoadChoice
  Matrix Concatenation1 : S-Function  FunctionName=smatrxcat  Parameters=numInports,catMethod  PortCounts=[]  SFunctionModules=''  mask(Matrix Concatenation){numInports=9, catMethod=Horizontal}
      mask prompts: numInports "Number of inputs:"; catMethod "Concatenation method:"
      mask help: Perform horizontal or vertical concatenation. 1-D vector input signals are treated as column vectors, i.e., [Mx1] matrices. The output is always a matrix.
      mask init:
      | xy = matrxcatmask('icon');
      mask StyleString: edit,popup(Horizontal|Vertical)
      mask Display:
      | plot(xy.x,xy.y);
      | text(0.15,0.86,xy.label);
  On12 : Constant  Value=vinf.AuxLoads.RadiatorCoolingFan.On
  Product11 : Product  Inputs=2  Multiplication=Element-wise(.*)  SaturateOnIntegerOverflow=on
  Subsystem9 : lib_cosimulation/Subsystem  ModelName='RadiatorCoolingFan'
  VehType : Constant  Value=vinf.AuxLoads.RadiatorCoolingFan.SaberVehType
  i1 : Constant  Value=vinf.AuxLoads.RadiatorCoolingFan.Data(1,2)
  i2 : Constant  Value=vinf.AuxLoads.RadiatorCoolingFan.Data(2,2)
  i3 : Constant  Value=vinf.AuxLoads.RadiatorCoolingFan.Data(3,2)
  v1 : Constant  Value=vinf.AuxLoads.RadiatorCoolingFan.Data(1,1)
  v2 : Constant  Value=vinf.AuxLoads.RadiatorCoolingFan.Data(2,1)
  v3 : Constant  Value=vinf.AuxLoads.RadiatorCoolingFan.Data(3,1)
  Out1 : Outport  Port=1
  wires:
  Matrix Concatenation1/1 -> Out1/1
  LoadChoice/1 -> Matrix Concatenation1/8
  i3/1 -> Matrix Concatenation1/7
  i2/1 -> Matrix Concatenation1/6
  i1/1 -> Matrix Concatenation1/5
  v3/1 -> Matrix Concatenation1/4
  v2/1 -> Matrix Concatenation1/3
  v1/1 -> Matrix Concatenation1/2
  VehType/1 -> Matrix Concatenation1/1
  Product11/1 -> Matrix Concatenation1/9
  On12/1 -> Product11/1
  Subsystem9/1 -> Product11/2

== system lib_cosimulation/Aux Loads 14V/Radio ==
  Matrix Concatenation1 : S-Function  FunctionName=smatrxcat  Parameters=numInports,catMethod  PortCounts=[]  SFunctionModules=''  mask(Matrix Concatenation){numInports=8, catMethod=Horizontal}
      mask prompts: numInports "Number of inputs:"; catMethod "Concatenation method:"
      mask help: Perform horizontal or vertical concatenation. 1-D vector input signals are treated as column vectors, i.e., [Mx1] matrices. The output is always a matrix.
      mask init:
      | xy = matrxcatmask('icon');
      mask StyleString: edit,popup(Horizontal|Vertical)
      mask Display:
      | plot(xy.x,xy.y);
      | text(0.15,0.86,xy.label);
  Num1 : Constant  Value=vinf.AuxLoads.Radio.Num
  On3 : Constant  Value=vinf.AuxLoads.Radio.On
  Product3 : Product  Inputs=3  Multiplication=Element-wise(.*)  SaturateOnIntegerOverflow=on
  Subsystem : lib_cosimulation/Subsystem  ModelName='Radio'
  VehType : Constant  Value=vinf.AuxLoads.Radio.SaberVehType
  i1 : Constant  Value=vinf.AuxLoads.Radio.Data(1,2)
  i2 : Constant  Value=vinf.AuxLoads.Radio.Data(2,2)
  i3 : Constant  Value=vinf.AuxLoads.Radio.Data(3,2)
  v1 : Constant  Value=vinf.AuxLoads.Radio.Data(1,1)
  v2 : Constant  Value=vinf.AuxLoads.Radio.Data(2,1)
  v3 : Constant  Value=vinf.AuxLoads.Radio.Data(3,1)
  Out1 : Outport  Port=1
  wires:
  i3/1 -> Matrix Concatenation1/7
  i2/1 -> Matrix Concatenation1/6
  i1/1 -> Matrix Concatenation1/5
  v3/1 -> Matrix Concatenation1/4
  v2/1 -> Matrix Concatenation1/3
  v1/1 -> Matrix Concatenation1/2
  VehType/1 -> Matrix Concatenation1/1
  Matrix Concatenation1/1 -> Out1/1
  Product3/1 -> Matrix Concatenation1/8
  Num1/1 -> Product3/2
  Subsystem/1 -> Product3/3
  On3/1 -> Product3/1

== system lib_cosimulation/Aux Loads 14V/RearDefrost ==
  Matrix Concatenation1 : S-Function  FunctionName=smatrxcat  Parameters=numInports,catMethod  PortCounts=[]  SFunctionModules=''  mask(Matrix Concatenation){numInports=8, catMethod=Horizontal}
      mask prompts: numInports "Number of inputs:"; catMethod "Concatenation method:"
      mask help: Perform horizontal or vertical concatenation. 1-D vector input signals are treated as column vectors, i.e., [Mx1] matrices. The output is always a matrix.
      mask init:
      | xy = matrxcatmask('icon');
      mask StyleString: edit,popup(Horizontal|Vertical)
      mask Display:
      | plot(xy.x,xy.y);
      | text(0.15,0.86,xy.label);
  On1 : Constant  Value=vinf.AuxLoads.RearDefrost.On
  Product1 : Product  Inputs=2  Multiplication=Element-wise(.*)  SaturateOnIntegerOverflow=on
  Subsystem5 : lib_cosimulation/Subsystem  ModelName='RearDefrost'
  VehType : Constant  Value=vinf.AuxLoads.RearDefrost.SaberVehType
  i1 : Constant  Value=vinf.AuxLoads.RearDefrost.Data(1,2)
  i2 : Constant  Value=vinf.AuxLoads.RearDefrost.Data(2,2)
  i3 : Constant  Value=vinf.AuxLoads.RearDefrost.Data(3,2)
  v1 : Constant  Value=vinf.AuxLoads.RearDefrost.Data(1,1)
  v2 : Constant  Value=vinf.AuxLoads.RearDefrost.Data(2,1)
  v3 : Constant  Value=vinf.AuxLoads.RearDefrost.Data(3,1)
  Out1 : Outport  Port=1
  wires:
  VehType/1 -> Matrix Concatenation1/1
  i3/1 -> Matrix Concatenation1/7
  i2/1 -> Matrix Concatenation1/6
  i1/1 -> Matrix Concatenation1/5
  v3/1 -> Matrix Concatenation1/4
  v2/1 -> Matrix Concatenation1/3
  v1/1 -> Matrix Concatenation1/2
  Matrix Concatenation1/1 -> Out1/1
  On1/1 -> Product1/1
  Subsystem5/1 -> Product1/2
  Product1/1 -> Matrix Concatenation1/8

== system lib_cosimulation/Aux Loads 14V/RearHVAC ==
  LoadChoice : Constant  Value=vinf.AuxLoads.RearHVAC.SaberLoadChoice
  Matrix Concatenation1 : S-Function  FunctionName=smatrxcat  Parameters=numInports,catMethod  PortCounts=[]  SFunctionModules=''  mask(Matrix Concatenation){numInports=9, catMethod=Horizontal}
      mask prompts: numInports "Number of inputs:"; catMethod "Concatenation method:"
      mask help: Perform horizontal or vertical concatenation. 1-D vector input signals are treated as column vectors, i.e., [Mx1] matrices. The output is always a matrix.
      mask init:
      | xy = matrxcatmask('icon');
      mask StyleString: edit,popup(Horizontal|Vertical)
      mask Display:
      | plot(xy.x,xy.y);
      | text(0.15,0.86,xy.label);
  On9 : Constant  Value=vinf.AuxLoads.RearHVAC.On
  Product8 : Product  Inputs=2  Multiplication=Element-wise(.*)  SaturateOnIntegerOverflow=on
  Subsystem7 : lib_cosimulation/Subsystem  ModelName='RearHVAC'
  VehType : Constant  Value=vinf.AuxLoads.RearHVAC.SaberVehType
  i1 : Constant  Value=vinf.AuxLoads.RearHVAC.Data(1,2)
  i2 : Constant  Value=vinf.AuxLoads.RearHVAC.Data(2,2)
  i3 : Constant  Value=vinf.AuxLoads.RearHVAC.Data(3,2)
  v1 : Constant  Value=vinf.AuxLoads.RearHVAC.Data(1,1)
  v2 : Constant  Value=vinf.AuxLoads.RearHVAC.Data(2,1)
  v3 : Constant  Value=vinf.AuxLoads.RearHVAC.Data(3,1)
  Out1 : Outport  Port=1
  wires:
  LoadChoice/1 -> Matrix Concatenation1/8
  i3/1 -> Matrix Concatenation1/7
  i2/1 -> Matrix Concatenation1/6
  i1/1 -> Matrix Concatenation1/5
  v3/1 -> Matrix Concatenation1/4
  v2/1 -> Matrix Concatenation1/3
  v1/1 -> Matrix Concatenation1/2
  Matrix Concatenation1/1 -> Out1/1
  VehType/1 -> Matrix Concatenation1/1
  On9/1 -> Product8/1
  Product8/1 -> Matrix Concatenation1/9
  Subsystem7/1 -> Product8/2

== system lib_cosimulation/Aux Loads 14V/RearWipers ==
  Matrix Concatenation1 : S-Function  FunctionName=smatrxcat  Parameters=numInports,catMethod  PortCounts=[]  SFunctionModules=''  mask(Matrix Concatenation){numInports=8, catMethod=Horizontal}
      mask prompts: numInports "Number of inputs:"; catMethod "Concatenation method:"
      mask help: Perform horizontal or vertical concatenation. 1-D vector input signals are treated as column vectors, i.e., [Mx1] matrices. The output is always a matrix.
      mask init:
      | xy = matrxcatmask('icon');
      mask StyleString: edit,popup(Horizontal|Vertical)
      mask Display:
      | plot(xy.x,xy.y);
      | text(0.15,0.86,xy.label);
  On4 : Constant  Value=vinf.AuxLoads.RearWipers.On
  Product4 : Product  Inputs=2  Multiplication=Element-wise(.*)  SaturateOnIntegerOverflow=on
  Subsystem1 : lib_cosimulation/Subsystem  ModelName='RearWipers'
  VehType : Constant  Value=vinf.AuxLoads.RearWipers.SaberVehType
  i1 : Constant  Value=vinf.AuxLoads.RearWipers.Data(1,2)
  i2 : Constant  Value=vinf.AuxLoads.RearWipers.Data(2,2)
  i3 : Constant  Value=vinf.AuxLoads.RearWipers.Data(3,2)
  v1 : Constant  Value=vinf.AuxLoads.RearWipers.Data(1,1)
  v2 : Constant  Value=vinf.AuxLoads.RearWipers.Data(2,1)
  v3 : Constant  Value=vinf.AuxLoads.RearWipers.Data(3,1)
  Out1 : Outport  Port=1
  wires:
  i3/1 -> Matrix Concatenation1/7
  i2/1 -> Matrix Concatenation1/6
  i1/1 -> Matrix Concatenation1/5
  v3/1 -> Matrix Concatenation1/4
  v2/1 -> Matrix Concatenation1/3
  v1/1 -> Matrix Concatenation1/2
  Matrix Concatenation1/1 -> Out1/1
  VehType/1 -> Matrix Concatenation1/1
  Product4/1 -> Matrix Concatenation1/8
  On4/1 -> Product4/1
  Subsystem1/1 -> Product4/2

== system lib_cosimulation/Aux Loads 14V/Starter ==
  Matrix Concatenation1 : S-Function  FunctionName=smatrxcat  Parameters=numInports,catMethod  PortCounts=[]  SFunctionModules=''  mask(Matrix Concatenation){numInports=3, catMethod=Horizontal}
      mask prompts: numInports "Number of inputs:"; catMethod "Concatenation method:"
      mask help: Perform horizontal or vertical concatenation. 1-D vector input signals are treated as column vectors, i.e., [Mx1] matrices. The output is always a matrix.
      mask init:
      | xy = matrxcatmask('icon');
      mask StyleString: edit,popup(Horizontal|Vertical)
      mask Display:
      | plot(xy.x,xy.y);
      | text(0.15,0.86,xy.label);
  On/Off : Gain  Gain=vinf.AuxLoadsOn  Multiplication=Element-wise(K.*u)  SaturateOnIntegerOverflow=on
  Product : Product  Inputs=2  Multiplication=Element-wise(.*)  SaturateOnIntegerOverflow=on
  Starter : Subsystem
      settings: RTWFcnNameOpts=Auto  RTWFileNameOpts=Auto
  VehType : Constant  Value=vinf.AuxLoads.Starter.DurationOn
  VehType1 : Constant  Value=(vinf.AuxLoads.Starter.Data*vinf.AuxLoads.Starter.V14)*14
  VehType3 : Constant  Value=vinf.AuxLoads.Starter.On
  Out1 : Outport  Port=1
  wires:
  VehType/1 -> Matrix Concatenation1/1
  Product/1 -> Matrix Concatenation1/2
  VehType1/1 -> Product/1
  VehType3/1 -> Product/2
  Matrix Concatenation1/1 -> Out1/1
  Starter/1(Starter_OnOff_Control) -> On/Off/1
  On/Off/1 -> Matrix Concatenation1/3
